simulink model "ejh57"  (Simulink 3.00)
settings: Solver=ode45  SolverMode=SingleTasking  StartTime=0.0  StopTime=5  FixedStep=0.01  RelTol=1e-3  AbsTol=1e-6
libraries: simulink3 x4
settings Model: OutputTimes=[1,2]  LastModifiedBy=Administrador

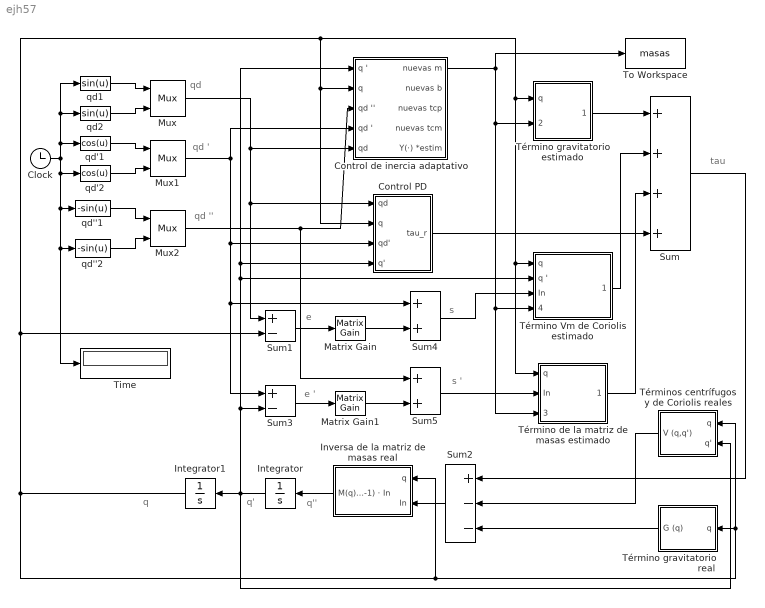
== system ejh57 ==
  note: q''
  note: q'
  note: q
  note: tau
  note: e
  note: e '
  note: s
  note: s '
  note: qd
  note: qd '
  note: qd ''
  Clock : Clock
      settings: DisplayTime=off  Decimation=10
  Control PD : Subsystem  mask(Controlador PD){A=[2.5 0;0 2.5], Kv=[10 0;0 10]}
      mask prompts: A "Introduzca la matriz A:"; Kv "Introduzca la matriz Kv:"
      mask help: Calcula el par tau_r correspondiente a la técnica del par computado usando un controlador PD.
  Control de inercia adaptativo : Subsystem  mask(Técnica del par computado con control adaptativo){dyn=[0 0 0 0 0 30 1 0 0 0 0 0 0 0 0 0 1 0 0 0;0 1 0 0 0 100 1 0 0 0 0 0 0 0 0 0 1 0 0 0], gamma=[20 0 zeros(1,6); 0 20 zeros(1,6); zeros(6,8)], a=[2.5 0;0 2.5], grav=[0 -9.81 0], m_inicial=[30 100], b_inicial=[0 0], tcp_inicial=[0 0], tcm_inicial=[0 0]}
      mask prompts: dyn "Matriz de parámetros cinemáticos y dinámicos:"; gamma "Matriz gamma:"; a "Matriz A:"; grav "Vector aceleración de la gravedad:"; m_inicial "Estimaciones de las masas:"; b_inicial "Estimaciones de las fricciones viscosas:"; tcp_inicial "Estimaciones de las fricciones de Coulomb (rotación +):"; tcm_inicial "Estimaciones de las fricciones de Coulomb (rotación -):"
  Integrator : Integrator  Orientation=left  ExternalReset=none  InitialConditionSource=internal  InitialCondition=[0;0]  LimitOutput=off  UpperSaturationLimit=inf  LowerSaturationLimit=-inf  ShowSaturationPort=off  ShowStatePort=off  AbsoluteTolerance=auto
  Integrator1 : Integrator  Orientation=left  ExternalReset=none  InitialConditionSource=internal  InitialCondition=[0; 0]  LimitOutput=off  UpperSaturationLimit=inf  LowerSaturationLimit=-inf  ShowSaturationPort=off  ShowStatePort=off  AbsoluteTolerance=auto
  Inversa de la matriz de masas real : Subsystem  Orientation=left  mask(Inversa de la matriz de masas){dyn=[0 0 0 0 0 0.8 1 0 0 0 0 0 0 0 0 0 1 0 0 0;0 1 0 0 0 2.3 1 0 0 0 0 0 0 0 0 0 1 0 0 0]}
      mask prompts: dyn "Matriz de parámetros cinemáticos y dinámicos:"
      mask help: Este bloque calcula el producto de la inversa de la matriz de masas por el vector columna In que se le pasa como entrada.
  Matrix Gain : simulink3/Math/Matrix Gain  K=[2.5 0;0 2.5]
  Matrix Gain1 : simulink3/Math/Matrix Gain  K=[2.5 0;0 2.5]
  Mux : Mux  Inputs=2
      settings: DisplayOption=none
  Mux1 : Mux  Inputs=2
      settings: DisplayOption=none
  Mux2 : Mux  Inputs=2
      settings: DisplayOption=none
  Sum : Sum  Inputs=++++  SaturateOnIntegerOverflow=on
  Sum1 : Sum  Inputs=+-  SaturateOnIntegerOverflow=on
  Sum2 : Sum  Orientation=left  Inputs=+--  SaturateOnIntegerOverflow=on
  Sum3 : Sum  Inputs=+-  SaturateOnIntegerOverflow=on
  Sum4 : Sum  Inputs=++  SaturateOnIntegerOverflow=on
  Sum5 : Sum  Inputs=++  SaturateOnIntegerOverflow=on
  Time : Display
      settings: Format=short
  To Workspace : ToWorkspace  VariableName=masas  SampleTime=-1  SaveFormat=Matrix
  Término gravitatorio estimado : Subsystem  mask(Término gravitatorio estimado){dyn=[0 0 0 0 0 30 1 0 0 0 0 0 0 0 0 0 1 0 0 0;0 1 0 0 0 100 1 0 0 0 0 0 0 0 0 0 1 0 0 0], grav=[0 -9.81 0]}
      mask prompts: dyn "Matriz inicial de parámetros cinemáticos y dinámicos:"; grav "Vector aceleración de la gravedad:"
      mask help: Este bloque calcula el par correspondiente al término gravitatorio. Dispone de una entrada para proporcionarle las estimaciones de las masas en cada instante.
      mask Display:
      | plot([0.05 0.95],[0.05 0.95])
      | plot([0.8 0.95],[0.7 0.95])
      | plot([0.7 0.95],[0.8 0.95])
  Término gravitatorio real : Subsystem  Orientation=left  mask(Término gravitatorio){dyn=[0 0 0 0 0 0.8 1 0 0 0 0 0 0 0 0 0 1 0 0 0;0 1 0 0 0 2.3 1 0 0 0 0 0 0 0 0 0 1 0 0 0], grav=[0 -9.81 0]}
      mask prompts: dyn "Matriz de parámetros cinemáticos y dinámicos:"; grav "Vector aceleración de la gravedad:"
      mask help: Este bloque calcula el par correspondiente al término gravitatorio.
  Término Vm de Coriolis estimado : Subsystem  mask(Término estimado asociado a la matriz de masas){dyn=[0 0 0 0 0 30 1 0 0 0 0 0 0 0 0 0 1 0 0 0;0 1 0 0 0 100 1 0 0 0 0 0 0 0 0 0 1 0 0 0]}
      mask prompts: dyn "Matriz inicial de parámetros cinemáticos y dinámicos:"
      mask help: Este bloque calcula el par correspondiente al término en el que aparece la matriz de masas. Dispone de una entrada para proporcionarle las estimaciones de las masas en cada instante.
      mask Display:
      | plot([0.05 0.95],[0.05 0.95])
      | plot([0.8 0.95],[0.7 0.95])
      | plot([0.7 0.95],[0.8 0.95])
  Término de la matriz de masas estimado : Subsystem  mask(Término estimado asociado a la matriz de masas){dyn=[0 0 0 0 0 30 1 0 0 0 0 0 0 0 0 0 1 0 0 0;0 1 0 0 0 100 1 0 0 0 0 0 0 0 0 0 1 0 0 0]}
      mask prompts: dyn "Matriz inicial de parámetros cinemáticos y dinámicos:"
      mask help: Este bloque calcula el par correspondiente al término en el que aparece la matriz de masas. Dispone de una entrada para proporcionarle las estimaciones de las masas en cada instante.
      mask Display:
      | plot([0.05 0.95],[0.05 0.95])
      | plot([0.8 0.95],[0.7 0.95])
      | plot([0.7 0.95],[0.8 0.95])
  Términos centrífugos y de Coriolis reales : Subsystem  Orientation=left  mask(Términos centrífugos y de Coriolis){dyn=[0 0 0 0 0 0.8 1 0 0 0 0 0 0 0 0 0 1 0 0 0;0 1 0 0 0 2.3 1 0 0 0 0 0 0 0 0 0 1 0 0 0]}
      mask prompts: dyn "Matriz de parámetros cinemáticos y dinámicos:"
      mask help: Este bloque calcula el par correspondiente a los términos centrífugos y de Coriolis.
  qd''1 : Fcn  Expr=-sin(u)
  qd''2 : Fcn  Expr=-sin(u)
  qd'1 : Fcn  Expr=cos(u)
  qd'2 : Fcn  Expr=cos(u)
  qd1 : Fcn  Expr=sin(u)
  qd2 : Fcn  Expr=sin(u)
  wires:
  qd''2/1 -> Mux2/2
  qd''1/1 -> Mux2/1
  qd'2/1 -> Mux1/2
  qd'1/1 -> Mux1/1
  qd2/1 -> Mux/2
  qd1/1 -> Mux/1
  Control PD/1(tau_r) -> Sum/4
  Término Vm de Coriolis estimado/1(Vm (q,q')·In) -> Sum/2
  Término de la matriz de masas estimado/1(M (q)·In) -> Sum/3
  Clock/1 -> qd''1/1, qd''2/1, Time/1, qd'2/1, qd'1/1, qd1/1, qd2/1
  Mux1/1 -> Control PD/3(qd'), Sum3/1, Sum4/1, Control de inercia adaptativo/4(qd ')
  Sum1/1 -> Matrix Gain/1
  Sum3/1 -> Matrix Gain1/1
  Matrix Gain1/1 -> Sum5/2
  Matrix Gain/1 -> Sum4/2
  Sum5/1 -> Término de la matriz de masas estimado/2(In)
  Sum4/1 -> Término Vm de Coriolis estimado/3(In)
  Término gravitatorio estimado/1(G (q)) -> Sum/1
  Integrator/1 -> Integrator1/1, Términos centrífugos y de Coriolis reales/2(q'), Control de inercia adaptativo/1(q '), Control PD/4(q'), Término Vm de Coriolis estimado/2(q '), Sum3/2
  Sum2/1 -> Inversa de la matriz de masas real/2(In)
  Integrator1/1 -> Inversa de la matriz de masas real/1(q), Términos centrífugos y de Coriolis reales/1(q), Término gravitatorio real/1(q), Sum1/2, Control PD/2(q), Control de inercia adaptativo/2(q), Término gravitatorio estimado/1(q), Término Vm de Coriolis estimado/1(q), Término de la matriz de masas estimado/1(q)
  Inversa de la matriz de masas real/1(M(q)^(-1) · In) -> Integrator/1
  Sum/1 -> Sum2/1
  Mux/1 -> Control de inercia adaptativo/5(qd), Sum1/1, Control PD/1(qd)
  Mux2/1 -> Control de inercia adaptativo/3(qd ''), Sum5/1
  Términos centrífugos y de Coriolis reales/1(V (q,q')) -> Sum2/2
  Término gravitatorio real/1(G (q)) -> Sum2/3
  Control de inercia adaptativo/1(nuevas m) -> Término gravitatorio estimado/2(nuevas m), Término de la matriz de masas estimado/3(nuevas m), Término Vm de Coriolis estimado/4(nuevas m), To Workspace/1

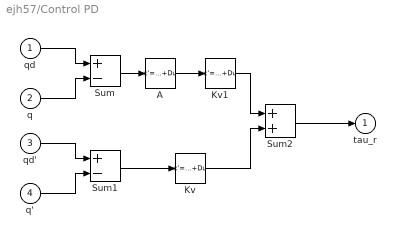
== system ejh57/Control PD ==
  qd : Inport  Port=1  PortWidth=-1  SampleTime=-1  DataType=auto
      settings: SignalType=auto
  q : Inport  Port=2  PortWidth=-1  SampleTime=-1  DataType=auto
      settings: SignalType=auto
  qd' : Inport  Port=3  PortWidth=-1  SampleTime=-1  DataType=auto
      settings: SignalType=auto
  q' : Inport  Port=4  PortWidth=-1  SampleTime=-1  DataType=auto
      settings: SignalType=auto
  A : StateSpace  A=[]  B=[]  C=[]  D=K  X0=0  mask(Matrix Gain){@1=A}
      mask prompts: @1 "Gain matrix:"
      mask help: Matrix Gain.
      mask init:
      | K=@1;
      mask Help: Multiplies input vector by entered matrix to produce output vector (y=Au).
      mask Display: disp('K')
  Kv : StateSpace  A=[]  B=[]  C=[]  D=K  X0=0  mask(Matrix Gain){@1=Kv}
      mask prompts: @1 "Gain matrix:"
      mask help: Matrix Gain.
      mask init:
      | K=@1;
      mask Help: Multiplies input vector by entered matrix to produce output vector (y=Au).
      mask Display: disp('K')
  Kv1 : StateSpace  A=[]  B=[]  C=[]  D=K  X0=0  mask(Matrix Gain){@1=Kv}
      mask prompts: @1 "Gain matrix:"
      mask help: Matrix Gain.
      mask init:
      | K=@1;
      mask Help: Multiplies input vector by entered matrix to produce output vector (y=Au).
      mask Display: disp('K')
  Sum : Sum  Inputs=+-  SaturateOnIntegerOverflow=on
  Sum1 : Sum  Inputs=+-  SaturateOnIntegerOverflow=on
  Sum2 : Sum  Inputs=++  SaturateOnIntegerOverflow=on
  tau_r : Outport  Port=1  InitialOutput=0
  wires:
  Sum2/1 -> tau_r/1
  Kv1/1 -> Sum2/1
  Kv/1 -> Sum2/2
  Sum1/1 -> Kv/1
  q'/1 -> Sum1/2
  qd'/1 -> Sum1/1
  q/1 -> Sum/2
  qd/1 -> Sum/1
  Sum/1 -> A/1
  A/1 -> Kv1/1

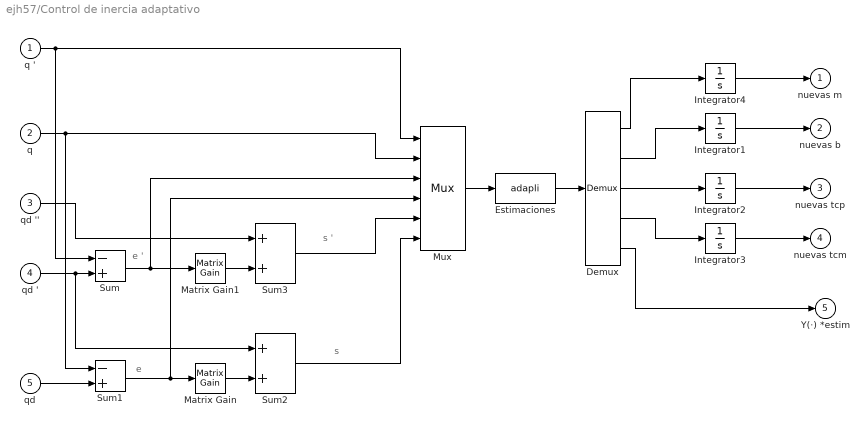
== system ejh57/Control de inercia adaptativo ==
  note: e
  note: e '
  note: s
  note: s '
  q ' : Inport  Port=1  PortWidth=-1  SampleTime=-1  DataType=auto
      settings: SignalType=auto
  q : Inport  Port=2  PortWidth=-1  SampleTime=-1  DataType=auto
      settings: SignalType=auto
  qd '' : Inport  Port=3  PortWidth=-1  SampleTime=-1  DataType=auto
      settings: SignalType=auto
  qd ' : Inport  Port=4  PortWidth=-1  SampleTime=-1  DataType=auto
      settings: SignalType=auto
  qd : Inport  Port=5  PortWidth=-1  SampleTime=-1  DataType=auto
      settings: SignalType=auto
  Demux : Demux  Outputs=5
  Estimaciones : S-Function  FunctionName=adapli  Parameters=dyn, gamma, a, grav  PortCounts=[]  SFunctionModules=''
  Integrator1 : Integrator  ExternalReset=none  InitialConditionSource=internal  InitialCondition=b_inicial(:)  LimitOutput=off  UpperSaturationLimit=inf  LowerSaturationLimit=-inf  ShowSaturationPort=off  ShowStatePort=off  AbsoluteTolerance=auto
  Integrator2 : Integrator  ExternalReset=none  InitialConditionSource=internal  InitialCondition=tcp_inicial(:)  LimitOutput=off  UpperSaturationLimit=inf  LowerSaturationLimit=-inf  ShowSaturationPort=off  ShowStatePort=off  AbsoluteTolerance=auto
  Integrator3 : Integrator  ExternalReset=none  InitialConditionSource=internal  InitialCondition=tcm_inicial(:)  LimitOutput=off  UpperSaturationLimit=inf  LowerSaturationLimit=-inf  ShowSaturationPort=off  ShowStatePort=off  AbsoluteTolerance=auto
  Integrator4 : Integrator  ExternalReset=none  InitialConditionSource=internal  InitialCondition=m_inicial(:)  LimitOutput=off  UpperSaturationLimit=inf  LowerSaturationLimit=-inf  ShowSaturationPort=off  ShowStatePort=off  AbsoluteTolerance=auto
  Matrix Gain : simulink3/Math/Matrix Gain  K=a
  Matrix Gain1 : simulink3/Math/Matrix Gain  K=a
  Mux : Mux  Inputs=6
      settings: DisplayOption=none
  Sum : Sum  Inputs=-+  SaturateOnIntegerOverflow=on
  Sum1 : Sum  Inputs=-+  SaturateOnIntegerOverflow=on
  Sum2 : Sum  Inputs=++  SaturateOnIntegerOverflow=on
  Sum3 : Sum  Inputs=++  SaturateOnIntegerOverflow=on
  nuevas m : Outport  Port=1  InitialOutput=0
  nuevas b : Outport  Port=2  InitialOutput=0
  nuevas tcp : Outport  Port=3  InitialOutput=0
  nuevas tcm : Outport  Port=4  InitialOutput=0
  Y(·) *estim : Outport  Port=5  InitialOutput=0
  wires:
  q '/1 -> Mux/1, Sum/1
  q/1 -> Mux/2, Sum1/1
  Mux/1 -> Estimaciones/1
  Estimaciones/1 -> Demux/1
  Demux/2 -> Integrator1/1
  Integrator1/1 -> nuevas b/1
  Demux/3 -> Integrator2/1
  Integrator2/1 -> nuevas tcp/1
  Demux/4 -> Integrator3/1
  Integrator3/1 -> nuevas tcm/1
  qd/1 -> Sum1/2
  Matrix Gain/1 -> Sum2/2
  qd '/1 -> Sum/2, Sum2/1
  Matrix Gain1/1 -> Sum3/2
  qd ''/1 -> Sum3/1
  Sum2/1 -> Mux/6
  Sum3/1 -> Mux/5
  Sum/1 -> Matrix Gain1/1, Mux/3
  Sum1/1 -> Matrix Gain/1, Mux/4
  Demux/5 -> Y(·) *estim/1
  Demux/1 -> Integrator4/1
  Integrator4/1 -> nuevas m/1

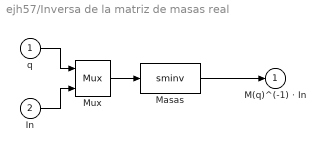
== system ejh57/Inversa de la matriz de masas real ==
  q : Inport  Port=1  PortWidth=-1  SampleTime=-1  DataType=auto
      settings: SignalType=auto
  In : Inport  Port=2  PortWidth=-1  SampleTime=-1  DataType=auto
      settings: SignalType=auto
  Masas : S-Function  FunctionName=sminv  Parameters=dyn  PortCounts=[]  SFunctionModules=''
  Mux : Mux  Inputs=2
      settings: DisplayOption=none
  M(q)^(-1) · In : Outport  Port=1  InitialOutput=0
  wires:
  Mux/1 -> Masas/1
  q/1 -> Mux/1
  In/1 -> Mux/2
  Masas/1 -> M(q)^(-1) · In/1

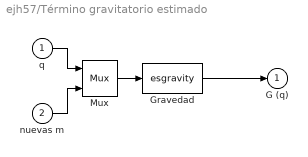
== system ejh57/Término gravitatorio estimado ==
  q : Inport  Port=1  PortWidth=-1  SampleTime=-1  DataType=auto
      settings: SignalType=auto
  nuevas m : Inport  Port=2  PortWidth=-1  SampleTime=-1  DataType=auto
      settings: SignalType=auto
  Gravedad : S-Function  FunctionName=esgravity  Parameters=dyn,grav  PortCounts=[]  SFunctionModules=''
  Mux : Mux  Inputs=2
      settings: DisplayOption=none
  G (q) : Outport  Port=1  InitialOutput=0
  wires:
  Mux/1 -> Gravedad/1
  nuevas m/1 -> Mux/2
  q/1 -> Mux/1
  Gravedad/1 -> G (q)/1

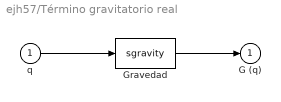
== system ejh57/Término gravitatorio real ==
  q : Inport  Port=1  PortWidth=-1  SampleTime=-1  DataType=auto
      settings: SignalType=auto
  Gravedad : S-Function  FunctionName=sgravity  Parameters=dyn,grav  PortCounts=[]  SFunctionModules=''
  G (q) : Outport  Port=1  InitialOutput=0
  wires:
  q/1 -> Gravedad/1
  Gravedad/1 -> G (q)/1

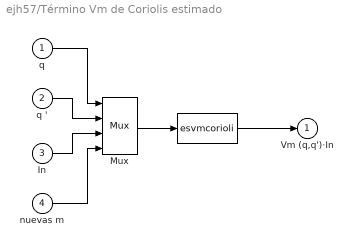
== system ejh57/Término Vm de Coriolis estimado ==
  q : Inport  Port=1  PortWidth=-1  SampleTime=-1  DataType=auto
      settings: SignalType=auto
  q ' : Inport  Port=2  PortWidth=-1  SampleTime=-1  DataType=auto
      settings: SignalType=auto
  In : Inport  Port=3  PortWidth=-1  SampleTime=-1  DataType=auto
      settings: SignalType=auto
  nuevas m : Inport  Port=4  PortWidth=-1  SampleTime=-1  DataType=auto
      settings: SignalType=auto
  "  " : S-Function  FunctionName=esvmcorioli  Parameters=dyn  PortCounts=[]  SFunctionModules=''
  Mux : Mux  Inputs=4
      settings: DisplayOption=none
  Vm (q,q')·In : Outport  Port=1  InitialOutput=0
  wires:
  nuevas m/1 -> Mux/4
  "  "/1 -> Vm (q,q')·In/1
  Mux/1 -> "  "/1
  In/1 -> Mux/3
  q/1 -> Mux/1
  q '/1 -> Mux/2

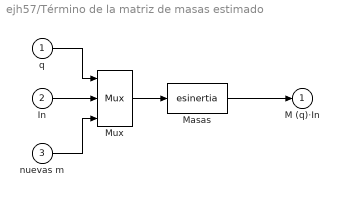
== system ejh57/Término de la matriz de masas estimado ==
  q : Inport  Port=1  PortWidth=-1  SampleTime=-1  DataType=auto
      settings: SignalType=auto
  In : Inport  Port=2  PortWidth=-1  SampleTime=-1  DataType=auto
      settings: SignalType=auto
  nuevas m : Inport  Port=3  PortWidth=-1  SampleTime=-1  DataType=auto
      settings: SignalType=auto
  Masas : S-Function  FunctionName=esinertia  Parameters=dyn  PortCounts=[]  SFunctionModules=''
  Mux : Mux  Inputs=3
      settings: DisplayOption=none
  M (q)·In : Outport  Port=1  InitialOutput=0
  wires:
  nuevas m/1 -> Mux/3
  Masas/1 -> M (q)·In/1
  Mux/1 -> Masas/1
  q/1 -> Mux/1
  In/1 -> Mux/2

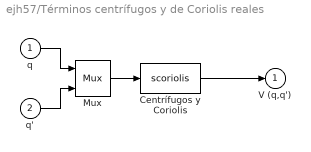
== system ejh57/Términos centrífugos y de Coriolis reales ==
  q : Inport  Port=1  PortWidth=-1  SampleTime=-1  DataType=auto
      settings: SignalType=auto
  q' : Inport  Port=2  PortWidth=-1  SampleTime=-1  DataType=auto
      settings: SignalType=auto
  Centrífugos y Coriolis : S-Function  FunctionName=scoriolis  Parameters=dyn  PortCounts=[]  SFunctionModules=''
  Mux : Mux  Inputs=2
      settings: DisplayOption=none
  V (q,q') : Outport  Port=1  InitialOutput=0
  wires:
  Mux/1 -> Centrífugos y Coriolis/1
  q/1 -> Mux/1
  q'/1 -> Mux/2
  Centrífugos y Coriolis/1 -> V (q,q')/1
